simulink model "project2"  (R2024a)
settings: Solver=VariableStepAuto  StartTime=0.0  StopTime=1690  RelTol=1e-3

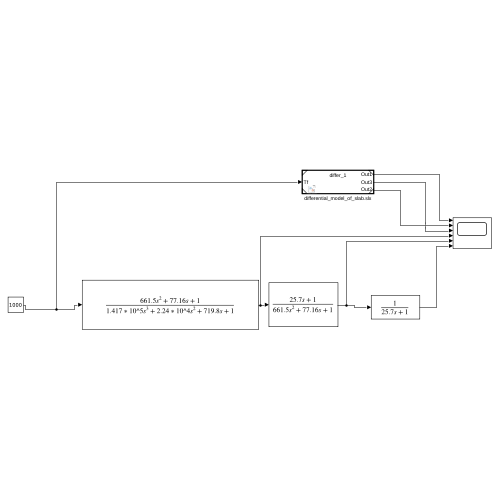
[thumbnail: Simulink's stored preview of the top-level diagram]
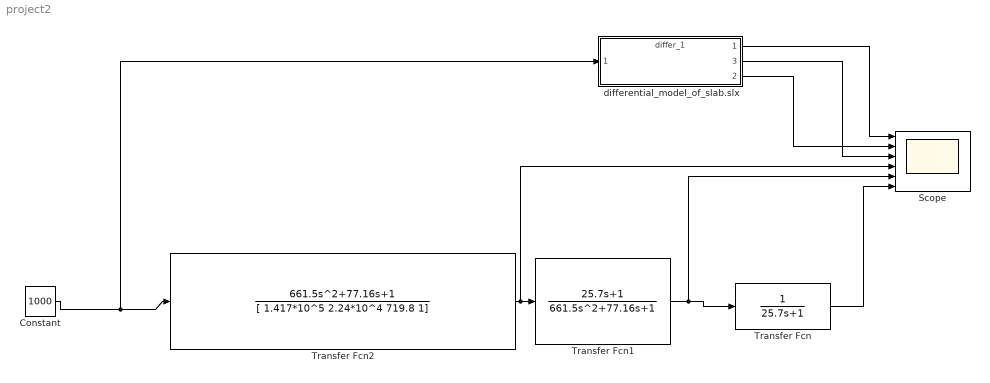
== system project2 ==
  Constant : Constant  Value=1000
  Scope : Scope  NumInputPorts=6
  Transfer Fcn : TransferFcn  Denominator=[25.7 1]
  Transfer Fcn1 : TransferFcn  Numerator=[25.7 1]  Denominator=[661.5 77.16 1]
  Transfer Fcn2 : TransferFcn  Numerator=[661.5 77.16 1]  Denominator=[ 1.417*10^5 2.24*10^4 719.8 1]
  differential_model_of_slab.slx : ModelReference  ModelNameDialog=differ_1.slx  SimulationMode=Normal  ModelReferenceVersion=1.3
      settings: PortSchema="{\"entries\":[{\"content\":{\"sides\":[{\"content\":{\"connectorIds\":[\"In1\"]},\"type\":\"ConnectorPlacement.EquallySpacedRectSide\",\"uuid\":\"1076a43c-205a-46e8-9d26-ce10804491d3\"},{\"content\":{\"connectorIds\":[\"Out1\",\"Out3\",\"Out2\"],\"side\":\"RIGHT\"},\"type\":\"ConnectorPlacement.EquallySpacedRectSide\",\"uuid\":\"291c2974-3192-4e9f-8569-70343557627b\"},{\"content\":{\"side\":\"TOP\"},\"type\":\"ConnectorPlacement.EquallySpacedRectSide\",\"uuid\":\"2d3dc940-b93b-449f-8646-58ea6faad965\"}]},\"type\":\"ConnectorPlacement.EquallySpacedConnector\",\"uuid\":\"92c42ed0-5e8b-4a3b-bcae-5216d415b6ff\"}],\"packageUris\":[\"http://schema.mathworks.com/mf0/Connector/R2020b\"],\"version\":\"1.0\"}"
  wires:
  Transfer Fcn1/1 -> Scope/5, Transfer Fcn/1
  Constant/1 -> differential_model_of_slab.slx/1, Transfer Fcn2/1
  Transfer Fcn/1 -> Scope/6
  Transfer Fcn2/1 -> Scope/4, Transfer Fcn1/1
  differential_model_of_slab.slx/3 -> Scope/3
  differential_model_of_slab.slx/2 -> Scope/2
  differential_model_of_slab.slx/1 -> Scope/1
